simulink model "W04_0_offline"  (R2024b)
settings: Solver=ode4  StartTime=0.0  StopTime=T_end  FixedStep=Ts  RelTol=1e-3
values from neighbouring files (symbols this model uses):
  gps_x = -0.85    [W04_setup.m]    (also in W09_setup.m)
  gps_y = 0.0    (= 0)    [W04_setup.m]    (also in W09_setup.m)
  half_beam = 1.027135    [W04_setup.m]    (also in W09_setup.m)
  hz_design_gps = 20    [W04_setup.m]    (also in W09_setup.m)
  hz_design_imu = 100    [W04_setup.m]    (also in W09_setup.m)
  imu_gyro_bias = 0.00075    [W04_setup.m]    (also in W09_setup.m)
  imu_gyro_std = 0.009    [W04_setup.m]    (also in W09_setup.m)
  imu_seed = 1    [W04_setup.m]    (also in W09_setup.m)
  Izz = 653    [W04_setup.m]    (also in W09_setup.m; build_w04_models.m = p(2); build_w09_models.m = p(2))
  lat0 = -33.72276870341191    (= -33.7227687034)    [W04_setup.m]    (also in W09_offline_run.m = evalin('base','lat0'); W09_setup.m)
  lon0 = 150.67399057896623    (= 150.673990579)    [W04_setup.m]    (also in W09_offline_run.m = evalin('base','lon0'); W09_setup.m)
  m_usv = 211    [W04_setup.m]    (also in W09_setup.m)
  Nr = 800    [W04_setup.m]    (also in W09_setup.m)
  Nrr = 800    [W04_setup.m]    (also in W09_setup.m; build_w04_models.m = p(8); build_w09_models.m = p(8))
  thrust_left = -200    [W04_setup.m]    (also in W09_setup.m)
  thrust_right = 200    [W04_setup.m]    (also in W09_setup.m)
  Ts = 0.005    [W04_setup.m]    (also in W09_offline_run.m = evalin('base','Ts'); W09_setup.m)
  x0_w04 = zeros(6,1)    [W04_setup.m]    (also in W09_setup.m)
  Xu = 100    [W04_setup.m]    (also in W09_setup.m; build_w04_models.m = p(3); build_w09_models.m = p(3))
  Xuu = 150    [W04_setup.m]    (also in W09_setup.m; build_w04_models.m = p(4); build_w09_models.m = p(4))
  Yv = 100    [W04_setup.m]    (also in W09_setup.m; build_w04_models.m = p(5); build_w09_models.m = p(5))
  Yvv = 100    [W04_setup.m]    (also in W09_setup.m; build_w04_models.m = p(6);'                newline  'Nr=p(7); build_w09_models.m = p(6);'                newline  'Nr=p(7))
settings Model: Creator=admin  LastModifiedBy=admin

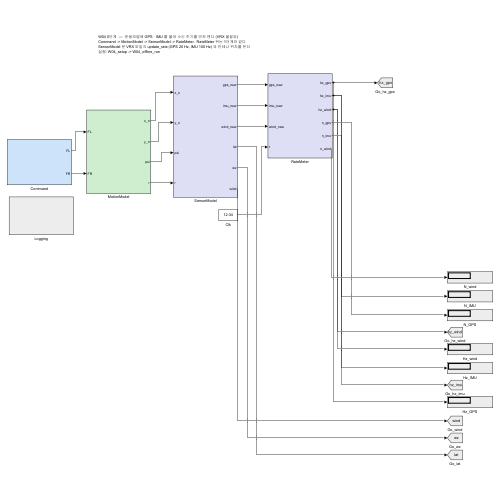
[thumbnail: Simulink's stored preview of the top-level diagram]
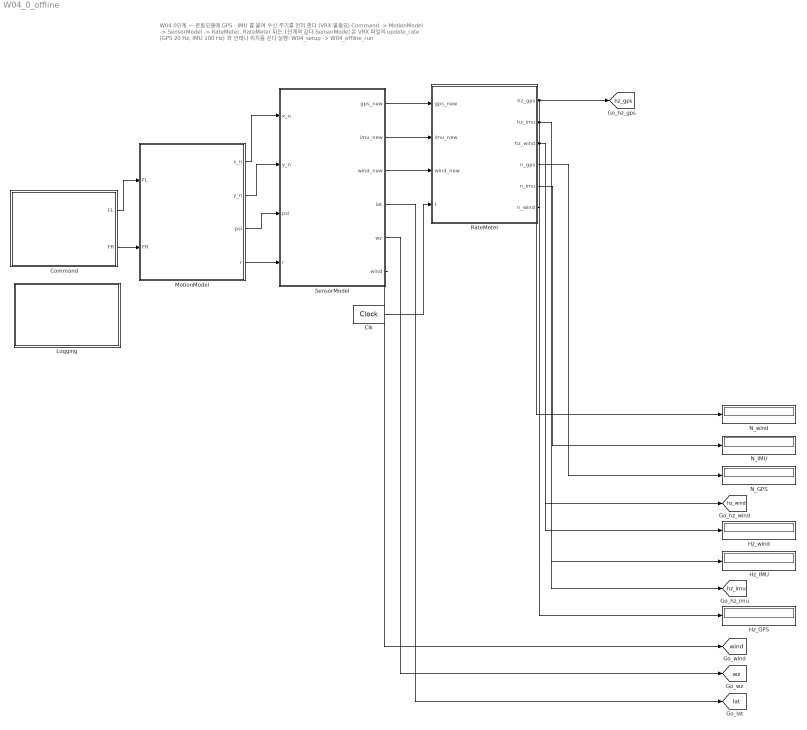
== system W04_0_offline ==
  note: W04 0단계  —  운동모델에 GPS · IMU 를 붙여 수신 주기를 먼저 잰다 (VRX 불필요)
      | Command -> MotionModel -> SensorModel -> RateMeter.  RateMeter 뒤는 1단계와 같다
      | SensorModel 은 VRX 파일의 update_rate (GPS 20 Hz, IMU 100 Hz) 와 안테나 위치를 쓴다
      | 실행: W04_setup -> W04_offline_run
  Clk : DigitalClock  SampleTime=Ts
  Command : Subsystem
  Hz_GPS : Display
  Hz_IMU : Display
  Hz_wind : Display
  Logging : Subsystem
  MotionModel : Subsystem
  N_GPS : Display
  N_IMU : Display
  N_wind : Display
  RateMeter : Subsystem
  SensorModel : Subsystem
  tag scope: hz_gps=global, hz_imu=global, hz_wind=global, lat=global, wind=global, wz=global
  wires:
  Command/1(FL) -> MotionModel/1(FL)
  SensorModel/1(gps_new) -> RateMeter/1(gps_new)
  MotionModel/1(x_n) -> SensorModel/1(x_n)
  Command/2(FR) -> MotionModel/2(FR)
  MotionModel/3(psi) -> SensorModel/3(psi)
  MotionModel/2(y_n) -> SensorModel/2(y_n)
  MotionModel/4(r) -> SensorModel/4(r)
  SensorModel/2(imu_new) -> RateMeter/2(imu_new)
  SensorModel/3(wind_new) -> RateMeter/3(wind_new)
  Clk/1 -> RateMeter/4(t)
  RateMeter/6(n_wind) -> N_wind/1
  RateMeter/5(n_imu) -> N_IMU/1
  RateMeter/4(n_gps) -> N_GPS/1
  SensorModel/6(wind) -> [wind]
  SensorModel/5(wz) -> [wz]
  SensorModel/4(lat) -> [lat]
  RateMeter/1(hz_gps) -> [hz_gps], Hz_GPS/1
  RateMeter/3(hz_wind) -> [hz_wind], Hz_wind/1
  RateMeter/2(hz_imu) -> [hz_imu], Hz_IMU/1

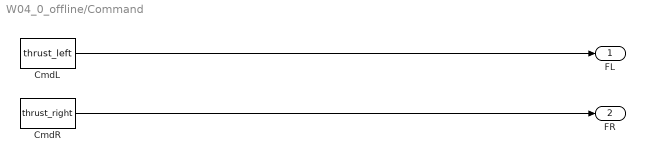
== system W04_0_offline/Command ==
  CmdL : Constant  Value=thrust_left
  CmdR : Constant  Value=thrust_right
  FL : Outport
  FR : Outport  Port=2
  wires:
  CmdL/1 -> FL/1
  CmdR/1 -> FR/1

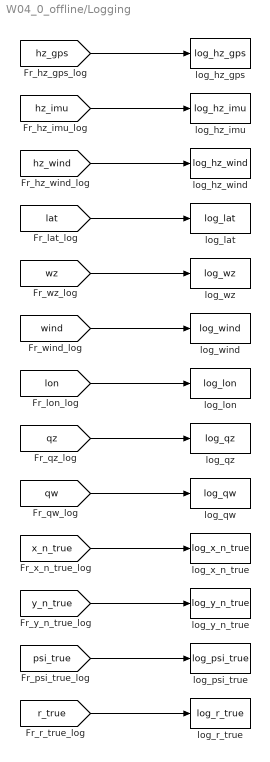
== system W04_0_offline/Logging ==
  log_hz_gps : ToWorkspace  VariableName=log_hz_gps  SaveFormat=Timeseries  SampleTime=Ts
  log_hz_imu : ToWorkspace  VariableName=log_hz_imu  SaveFormat=Timeseries  SampleTime=Ts
  log_hz_wind : ToWorkspace  VariableName=log_hz_wind  SaveFormat=Timeseries  SampleTime=Ts
  log_lat : ToWorkspace  VariableName=log_lat  SaveFormat=Timeseries  SampleTime=Ts
  log_lon : ToWorkspace  VariableName=log_lon  SaveFormat=Timeseries  SampleTime=Ts
  log_psi_true : ToWorkspace  VariableName=log_psi_true  SaveFormat=Timeseries  SampleTime=Ts
  log_qw : ToWorkspace  VariableName=log_qw  SaveFormat=Timeseries  SampleTime=Ts
  log_qz : ToWorkspace  VariableName=log_qz  SaveFormat=Timeseries  SampleTime=Ts
  log_r_true : ToWorkspace  VariableName=log_r_true  SaveFormat=Timeseries  SampleTime=Ts
  log_wind : ToWorkspace  VariableName=log_wind  SaveFormat=Timeseries  SampleTime=Ts
  log_wz : ToWorkspace  VariableName=log_wz  SaveFormat=Timeseries  SampleTime=Ts
  log_x_n_true : ToWorkspace  VariableName=log_x_n_true  SaveFormat=Timeseries  SampleTime=Ts
  log_y_n_true : ToWorkspace  VariableName=log_y_n_true  SaveFormat=Timeseries  SampleTime=Ts
  wires:
  [hz_gps] -> log_hz_gps/1
  [hz_imu] -> log_hz_imu/1
  [hz_wind] -> log_hz_wind/1
  [lat] -> log_lat/1
  [wz] -> log_wz/1
  [wind] -> log_wind/1
  [lon] -> log_lon/1
  [qz] -> log_qz/1
  [qw] -> log_qw/1
  [x_n_true] -> log_x_n_true/1
  [y_n_true] -> log_y_n_true/1
  [psi_true] -> log_psi_true/1
  [r_true] -> log_r_true/1

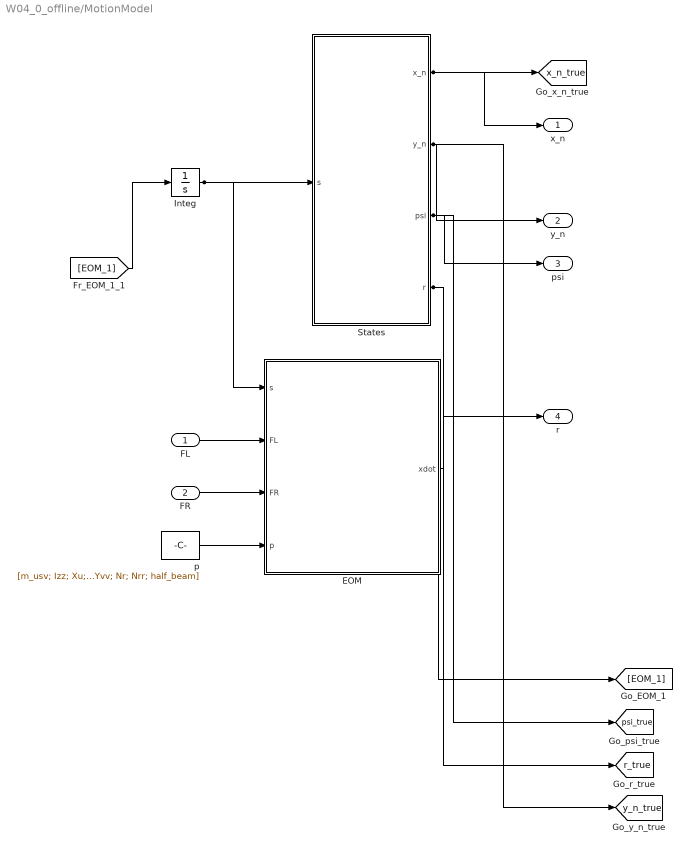
== system W04_0_offline/MotionModel ==
  FL : Inport
  FR : Inport  Port=2
  EOM : MATLAB Function  TreatAsAtomicUnit=on
  Integ : Integrator  InitialCondition=x0_w04
  States : MATLAB Function  TreatAsAtomicUnit=on
  p : Constant  Value=[m_usv; Izz; Xu; Xuu; Yv; Yvv; Nr; Nrr; half_beam]
  x_n : Outport
  y_n : Outport  Port=2
  psi : Outport  Port=3
  r : Outport  Port=4
  tag scope: psi_true=global, r_true=global, x_n_true=global, y_n_true=global
  wires:
  States/1(x_n) -> x_n/1, [x_n_true]
  p/1 -> EOM/4(p)
  Integ/1 -> States/1(s), EOM/1(s)
  FR/1 -> EOM/3(FR)
  FL/1 -> EOM/2(FL)
  States/2(y_n) -> y_n/1, [y_n_true]
  States/3(psi) -> psi/1, [psi_true]
  [EOM_1] -> Integ/1
  EOM/1(xdot) -> [EOM_1]
  States/4(r) -> [r_true], r/1

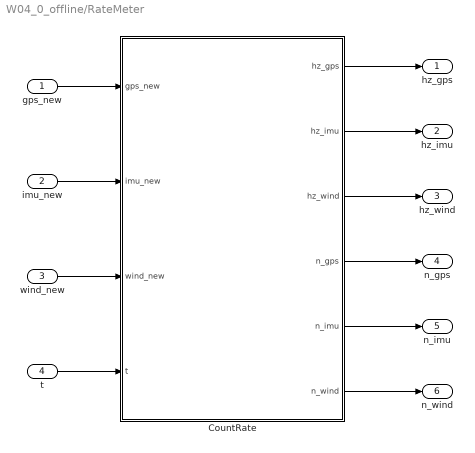
== system W04_0_offline/RateMeter ==
  gps_new : Inport
  imu_new : Inport  Port=2
  wind_new : Inport  Port=3
  t : Inport  Port=4
  CountRate : MATLAB Function  TreatAsAtomicUnit=on
  hz_gps : Outport
  hz_imu : Outport  Port=2
  hz_wind : Outport  Port=3
  n_gps : Outport  Port=4
  n_imu : Outport  Port=5
  n_wind : Outport  Port=6
  wires:
  gps_new/1 -> CountRate/1(gps_new)
  imu_new/1 -> CountRate/2(imu_new)
  CountRate/5(n_imu) -> n_imu/1
  CountRate/3(hz_wind) -> hz_wind/1
  CountRate/2(hz_imu) -> hz_imu/1
  wind_new/1 -> CountRate/3(wind_new)
  t/1 -> CountRate/4(t)
  CountRate/1(hz_gps) -> hz_gps/1
  CountRate/4(n_gps) -> n_gps/1
  CountRate/6(n_wind) -> n_wind/1

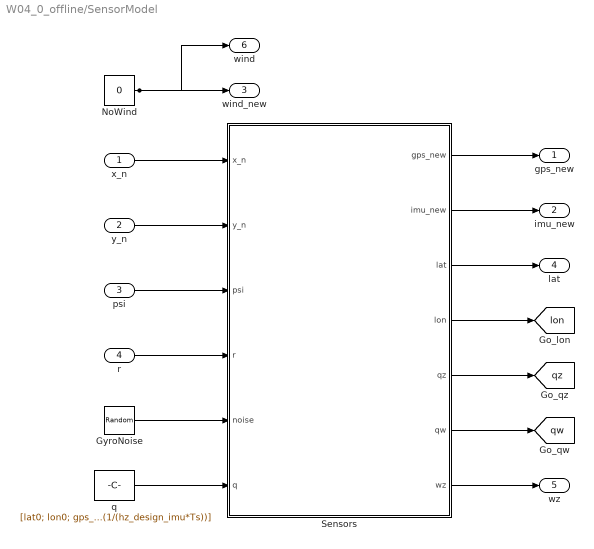
== system W04_0_offline/SensorModel ==
  x_n : Inport
  y_n : Inport  Port=2
  psi : Inport  Port=3
  r : Inport  Port=4
  GyroNoise : RandomNumber  Variance=imu_gyro_std^2  Seed=imu_seed  SampleTime=Ts
  NoWind : Constant  Value=0
  Sensors : MATLAB Function  TreatAsAtomicUnit=on
  q : Constant  Value=[lat0; lon0; gps_x; gps_y; imu_gyro_bias; round(1/(hz_design_gps*Ts)); round(1/(hz_design_imu*Ts))]
  gps_new : Outport
  imu_new : Outport  Port=2
  wind_new : Outport  Port=3
  lat : Outport  Port=4
  wz : Outport  Port=5
  wind : Outport  Port=6
  tag scope: lon=global, qw=global, qz=global
  wires:
  psi/1 -> Sensors/3(psi)
  NoWind/1 -> wind_new/1, wind/1
  x_n/1 -> Sensors/1(x_n)
  q/1 -> Sensors/6(q)
  r/1 -> Sensors/4(r)
  y_n/1 -> Sensors/2(y_n)
  GyroNoise/1 -> Sensors/5(noise)
  Sensors/5(qz) -> [qz]
  Sensors/3(lat) -> lat/1
  Sensors/1(gps_new) -> gps_new/1
  Sensors/4(lon) -> [lon]
  Sensors/2(imu_new) -> imu_new/1
  Sensors/6(qw) -> [qw]
  Sensors/7(wz) -> wz/1

== matlab function W04_0_offline/MotionModel/States ==
  data: s input; x_n output; y_n output; psi output; r output
function [x_n, y_n, psi, r] = States(s)
%#codegen
% 상태 벡터 s = [u v r x_n y_n psi] 에서 센서 모델이 쓰는 네 개를 꺼낸다.
r = s(3);
x_n = s(4);  y_n = s(5);
psi = atan2(sin(s(6)), cos(s(6)));

== matlab function W04_0_offline/MotionModel/EOM ==
  data: s input; xdot output; FL input; FR input; p input
function xdot = EOM(s, FL, FR, p)
%#codegen
% 3-DOF WAM-V equations of motion, NED.
% Coefficients come straight from the Gazebo VRX plugins.
%   s = [u v r x_n y_n psi]'
%   p = [m Izz Xu Xuu Yv Yvv Nr Nrr half_beam]'
u = s(1); v = s(2); r = s(3); psi = s(6);
m=p(1); Izz=p(2); Xu=p(3); Xuu=p(4); Yv=p(5); Yvv=p(6);
Nr=p(7); Nrr=p(8); b_half=p(9);

X = FL + FR;
N = (FL - FR)*b_half;

Dx = (Xu + Xuu*abs(u))*u;
Dy = (Yv + Yvv*abs(v))*v;
Dn = (Nr + Nrr*abs(r))*r;

du = (X - Dx)/m + v*r;
dv = (  - Dy)/m - u*r;
dr = (N - Dn)/Izz;

xdot = [du; dv; dr;
        u*cos(psi) - v*sin(psi);
        u*sin(psi) + v*cos(psi);
        r];

== matlab function W04_0_offline/SensorModel/Sensors ==
  settings: updateMethod=DISCRETE  sampleTime=Ts
  data: x_n input; gps_new output; y_n input; psi input; r input; noise input; q input; imu_new output; lat output; lon output; qz output; qw output; wz output
function [gps_new, imu_new, lat, lon, qz, qw, wz] = Sensors(x_n, y_n, psi, r, noise, q)
%#codegen
% GPS 와 IMU 를 VRX 처럼 흉내 낸다 (4주차 1-5 절).
%   GPS : 안테나 위치(선체 x = gps_x)의 위경도. nG 스텝마다 한 번 새 값
%   IMU : ENU 쿼터니언과 z 각속도(ENU, 잡음 + 바이어스). nI 스텝마다 한 번
%   q = [lat0 lon0 gps_x gps_y bias nG nI]'
persistent k lat_h lon_h qz_h qw_h wz_h
if isempty(k)
    k = 0;  lat_h = q(1);  lon_h = q(2);  qz_h = 0;  qw_h = 1;  wz_h = 0;
end
% 안테나 위치 — 선체 원점에서 (gps_x, gps_y) 만큼 떨어진 점 (3주차 1-5 회전)
xa = x_n + q(3)*cos(psi) - q(4)*sin(psi);
ya = y_n + q(3)*sin(psi) + q(4)*cos(psi);
% NED -> 위경도 (3주차 1-5 식의 역변환, WGS84)
a = 6378137.0;  e2 = 6.69437999014e-3;
lat0r = q(1)*pi/180;  s2 = sin(lat0r)^2;
Rm = a*(1 - e2)/(1 - e2*s2)^1.5;  Rn = a/sqrt(1 - e2*s2);
gps_new = double(mod(k, q(6)) == 0);
if gps_new > 0
    lat_h = q(1) + xa/Rm*180/pi;
    lon_h = q(2) + ya/(Rn*cos(lat0r))*180/pi;
end
imu_new = double(mod(k, q(7)) == 0);
if imu_new > 0
    yaw = pi/2 - psi;                 % NED 선수각 -> ENU yaw
    qz_h = sin(yaw/2);  qw_h = cos(yaw/2);
    wz_h = -r + q(5) + noise;         % r_ENU = -r_NED, 잡음 + 바이어스
end
k = k + 1;
lat = lat_h;  lon = lon_h;  qz = qz_h;  qw = qw_h;  wz = wz_h;

== matlab function W04_0_offline/RateMeter/CountRate ==
  data: gps_new input; hz_gps output; imu_new input; wind_new input; t input; hz_imu output; hz_wind output; n_gps output; n_imu output; n_wind output
function [hz_gps, hz_imu, hz_wind, n_gps, n_imu, n_wind] = CountRate(gps_new, imu_new, wind_new, t)
%#codegen
% Count how many messages arrived and divide by elapsed time.
% This is what `ros2 topic hz` does, on the same wall clock.
persistent cg ci cw
if isempty(cg), cg = 0; ci = 0; cw = 0; end
if gps_new,  cg = cg + 1; end
if imu_new,  ci = ci + 1; end
if wind_new, cw = cw + 1; end

n_gps = cg;  n_imu = ci;  n_wind = cw;
if t > 0
    hz_gps = cg/t;  hz_imu = ci/t;  hz_wind = cw/t;
else
    hz_gps = 0;     hz_imu = 0;     hz_wind = 0;
end
